simulink model "W1P8"  (R2020b)
settings: Solver=VariableStepAuto  StartTime=0.0  StopTime=5  RelTol=1e-3
settings Model: EnablePacing=on  PacingRate=0.560000  Creator=saadh  LastModifiedBy=saadh

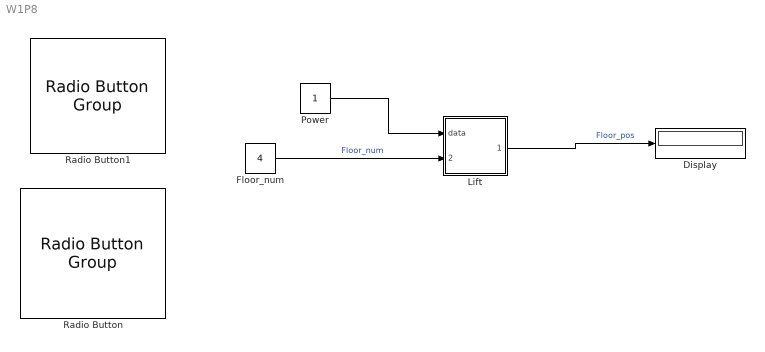
== system W1P8 ==
  Display : Display
  Floor_num : Constant  Value=4
  Lift : Stateflow chart  TreatAsAtomicUnit=on
  Power : Constant
  Radio Button : RadioButtonGroup  SelectedLabel=4th floor  ButtonGroupName=Group
      settings: Values={{'1st floor', '2nd floor', '3rd floor', '4th floor', '5th floor'}, [1 2 3 4 5]}
  Radio Button1 : RadioButtonGroup  SelectedLabel=PowerOn  ButtonGroupName=Group
      settings: Values={{'PowerOff', 'PowerOn'}, [0 1]}
  wires:
  Floor_num/1 -> Lift/2(Floor_num)  "Floor_num"
  Lift/1(Floor_pos) -> Display/1  "Floor_pos"
  Power/1 -> Lift/1(data)

== stateflow chart W1P8/Lift ==
  state PowerOn
    state Lift
      (history)
      state Floor5
        (history)
        state Dooropen1
          en:time=1;
          du:time = time+1;
        state Doorclose1
          en:time=1;
        (default) -> Dooropen1
        Dooropen1 -> Doorclose1 : [time==10]
      state Floor4
        (history)
        state Dooropen
          en:time=1;
          du:time = time+1;
        state Doorclose
          en:time=1;
        (default) -> PowerOn.Lift.Floor4.Dooropen
        PowerOn.Lift.Floor4.Dooropen -> PowerOn.Lift.Floor4.Doorclose : [time==10]
      state Floor3
        (history)
        state Dooropen
          en:time=1;
          du:time = time+1;
        state Doorclose
          en:time=1;
        (default) -> PowerOn.Lift.Floor3.Dooropen
        PowerOn.Lift.Floor3.Dooropen -> PowerOn.Lift.Floor3.Doorclose : [time==10]
      state Floor2
        (history)
        state Dooropen
          en:time=1;
          du:time = time+1;
        state Doorclose
          en:time=1;
        (default) -> PowerOn.Lift.Floor2.Dooropen
        PowerOn.Lift.Floor2.Dooropen -> PowerOn.Lift.Floor2.Doorclose : [time==10]
      state Floor1
        en:
        Floor_pos=1;
        (history)
        state Dooropen
          en:time=1;
          du:time = time+1;
        state Doorclose
          en:time=1;
        (default) -> PowerOn.Lift.Floor1.Dooropen
        PowerOn.Lift.Floor1.Dooropen -> PowerOn.Lift.Floor1.Doorclose : [time==10]
      Floor4 -> Floor5 [order 1] : [Floor_num>4]
      Floor5 -> Floor4 : [Floor_num<5]
      Floor3 -> Floor4 [order 1] : [Floor_num>3]
      Floor4 -> Floor3 [order 2] : [Floor_num<4]
      Floor2 -> Floor3 [order 1] : [Floor_num>2]
      Floor3 -> Floor2 [order 2] : [Floor_num<3]
      Floor1 -> Floor2 : [Floor_num>1]
      Floor2 -> Floor1 [order 2] : [Floor_num<2]
      (default) -> Floor1
    (default) -> Lift
  state PowerOff
  (default) -> PowerOff
  PowerOff -> PowerOn : [Power==1]
  PowerOn -> PowerOff : [Power==0]
  data: data input; Floor_num input; time local; Floor_pos output
